simulink model "F16_NzCAS"  (R2018b)
settings: Solver=ode4  StartTime=0.0  StopTime=10.0  FixedStep=0.01  RelTol=1e-3
values from neighbouring files (symbols this model uses):
  U_eq = [0.138585425211 -0.758630883044 1.0328691715e-16 -6.58183224618e-16]    [trim_data.mat]
undefined symbols (not defined in the file or in its folder): aircraft, k_p, k_q, nzP_eq, sigbuilder_block, tau_a, tau_e, tau_r, U0, X0, z
settings Model: Creator=rb3ir  LastModifiedBy=rb3ir
settings DataIOCC: SaveState=on

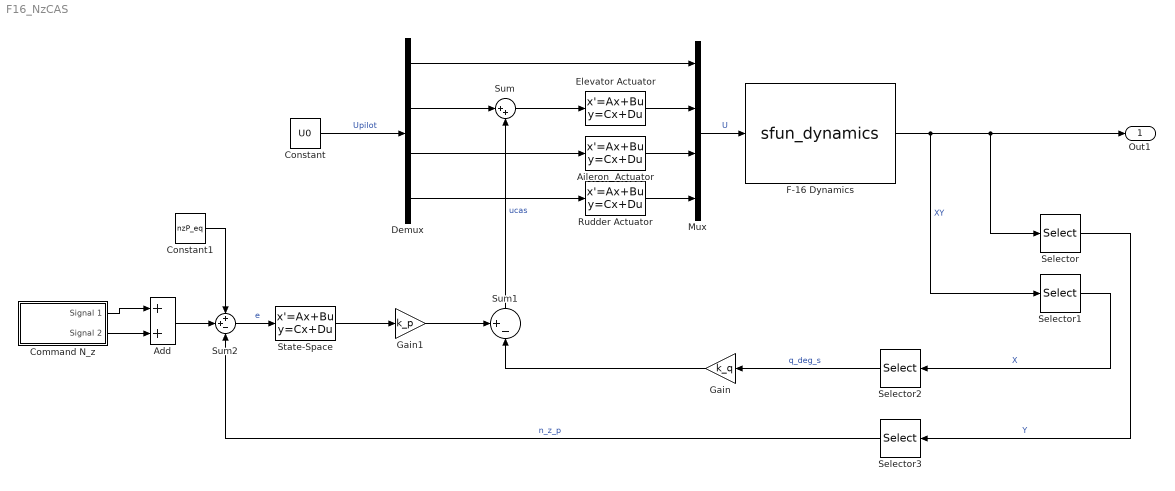
== system F16_NzCAS ==
  Add : Sum
  Aileron  Actuator : StateSpace  A=-1/tau_a  B=1/tau_a  D=0  InitialCondition=U_eq(3)
  Command N_z : Subsystem  Tag=STV Subsys  LoadFcn=sigbuilder_block('load');  StartFcn=sigbuilder_block('start');  StopFcn=sigbuilder_block('stop');  ClipboardFcn=sigbuilder_block('clipboard');  mask(Sigbuilder block){tuvar=[0:10]}
      mask help: Simulink:masks:SigbuilderBlock_MD
      mask init:
      | if ~strcmp(get_param(bdroot(gcbh),'SimulationStatus'),'stopped') tuvar = sigbuilder_block('maskInit'); end
      settings: CopyFcn=sigbuilder_block('copy');  DeleteFcn=sigbuilder_block('delete');  ModelCloseFcn=sigbuilder_block('modelClose');  PreSaveFcn=sigbuilder_block('preSave');  PauseFcn=sigbuilder_block('pause');  ContinueFcn=sigbuilder_block('continue');  NameChangeFcn=sigbuilder_block('namechange');  OpenFcn=sigbuilder_block('open',[437.6 153 550.4 359.25 ]);  CloseFcn=sigbuilder_block('close');
      mask Display: plot(0, 0, 100, 100,[2, 2, 32, 32, 2], [68, 8, 8, 68, 68],[32, 2], [38, 38], [32, 19, 2],[53, 60, 44], [32, 17, 17, 2],[16, 16, 31, 31]);txt = getActiveGroup(gcbh);text(2, 100, txt,'verticalAlignment', 'top');
  Constant : Constant  Value=U0
  Constant1 : Constant  Value=nzP_eq
  Demux : Demux
  Elevator Actuator : StateSpace  A=-1/tau_e  B=1/tau_e  D=0  InitialCondition=U_eq(2)
  F-16 Dynamics : S-Function  FunctionName=sfun_dynamics  Parameters=aircraft,X0  SFunctionDeploymentMode=off  EnableBusSupport=off
  Gain : Gain  Gain=k_q
  Gain1 : Gain  Gain=k_p
  Mux : Mux
  Rudder Actuator : StateSpace  A=-1/tau_r  B=1/tau_r  D=0  InitialCondition=U_eq(4)
  Selector : Selector  InputPortWidth=34  IndexOptions=Index vector (dialog)  Indices=[14:34]  OutputSizes=1
  Selector1 : Selector  InputPortWidth=34  IndexOptions=Index vector (dialog)  Indices=[1:13]  OutputSizes=1
  Selector2 : Selector  InputPortWidth=13  IndexOptions=Index vector (dialog)  Indices=[3]  OutputSizes=1
  Selector3 : Selector  InputPortWidth=21  IndexOptions=Index vector (dialog)  Indices=[21]  OutputSizes=1
  State-Space : StateSpace  A=0  B=z  InitialCondition=0
  Sum : Sum  Inputs=|++
  Sum1 : Sum  Inputs=+-|
  Sum2 : Sum  Inputs=++-
  Out1 : Outport
  wires:
  F-16 Dynamics/1 -> Out1/1, Selector/1, Selector1/1  "XY"
  Elevator Actuator/1 -> Mux/2
  Aileron  Actuator/1 -> Mux/3
  Rudder Actuator/1 -> Mux/4
  Mux/1 -> F-16 Dynamics/1  "U"
  Sum/1 -> Elevator Actuator/1
  Demux/1 -> Mux/1
  Demux/2 -> Sum/1
  Demux/3 -> Aileron  Actuator/1
  Demux/4 -> Rudder Actuator/1
  Constant/1 -> Demux/1  "Upilot"
  Selector/1 -> Selector3/1  "Y"
  Selector1/1 -> Selector2/1  "X"
  Selector2/1 -> Gain/1  "q_deg_s"
  Selector3/1 -> Sum2/3  "n_z_p"
  Gain/1 -> Sum1/2
  Sum1/1 -> Sum/2  "ucas"
  Sum2/1 -> State-Space/1  "e"
  State-Space/1 -> Gain1/1
  Gain1/1 -> Sum1/1
  Command N_z/1(Signal 1) -> Add/1
  Command N_z/2(Signal 2) -> Add/2
  Add/1 -> Sum2/2
  Constant1/1 -> Sum2/1

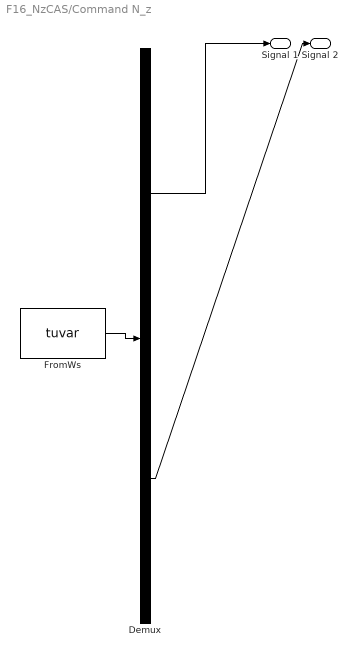
== system F16_NzCAS/Command N_z ==
  Demux : Demux  Tag=STV Demux  Outputs=2
  FromWs : FromWorkspace  Tag=STV FromWs  VariableName=tuvar  SampleTime=0
      SigBuilderData=|
      | common.afterFinalStr = 'Extrapolate'
      | common.sampleTime = 0
      | dataSet.timeRange = [0 30]
      | dataSet.name = 'Group 1'
      | sbobj.Groups.Name = 'Group 1'
      | sbobj.Groups.Signals(1).Name = 'Signal 1'
      | sbobj.Groups.Signals(1).XData = [0 1 1 11 11 30]
      | sbobj.Groups.Signals(1).YData = [0 0 1 1 0 0]
      | sbobj.Groups.Signals(2).Name = 'Signal 2'
      | sbobj.Groups.Signals(2).XData = [0 11 11 21 21 30]
      | sbobj.Groups.Signals(2).YData = [0 0 -1 -1 0 0]
      | sbobj.Groups.TimeRange = [0 30]
  Signal 1 : Outport  Tag=STV Outport
  Signal 2 : Outport  Tag=STV Outport  Port=2
  wires:
  Demux/1 -> Signal 1/1
  FromWs/1 -> Demux/1
  Demux/2 -> Signal 2/1
